simulink model "task1"  (R2024a)
settings: Solver=VariableStepAuto  StartTime=0.0  StopTime=10.0  MaxStep=0.01  RelTol=1e-3
undefined symbols (not defined in the file): A, B, Bf, CZ, G, K1, K2, wf0, x0
settings Model: Creator=sizgr  LastModifiedBy=sizgr

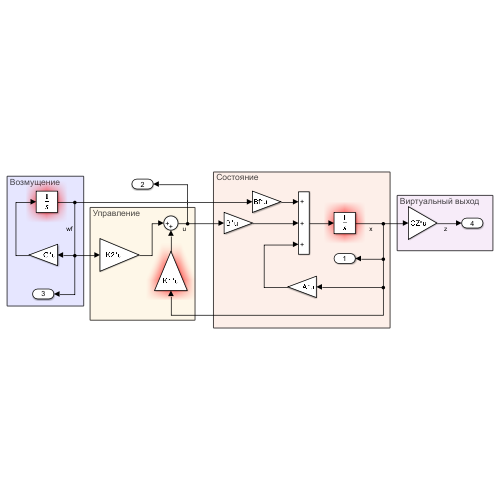
[thumbnail: Simulink's stored preview of the top-level diagram]
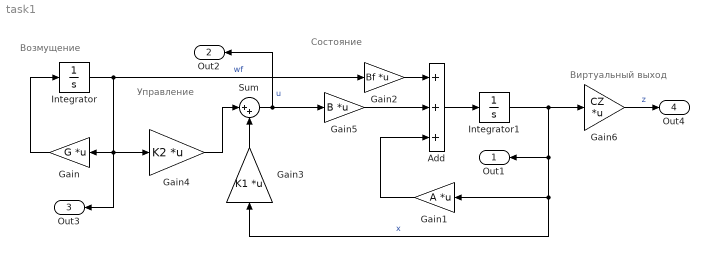
== system task1 ==
  note: Состояние
  note: Виртуальный выход
  note: Управление
  note: Возмущение
  Add : Sum  Inputs=+++
  Gain : Gain  Gain=G  Multiplication=Matrix(K*u)
  Gain1 : Gain  Gain=A  Multiplication=Matrix(K*u)
  Gain2 : Gain  Gain=Bf  Multiplication=Matrix(K*u)
  Gain3 : Gain  Gain=K1  Multiplication=Matrix(K*u)
  Gain4 : Gain  Gain=K2  Multiplication=Matrix(K*u)
  Gain5 : Gain  Gain=B  Multiplication=Matrix(K*u)
  Gain6 : Gain  Gain=CZ  Multiplication=Matrix(K*u)
  Integrator : Integrator  InitialCondition=wf0
  Integrator1 : Integrator  InitialCondition=x0
  Sum : Sum  Inputs=|++
  Out1 : Outport
  Out2 : Outport  Port=2
  Out3 : Outport  Port=3
  Out4 : Outport  Port=4
  wires:
  Integrator/1 -> Out3/1, Gain/1, Gain4/1, Gain2/1  "wf"
  Gain/1 -> Integrator/1
  Integrator1/1 -> Out1/1, Gain1/1, Gain3/1, Gain6/1  "x"
  Gain1/1 -> Add/3
  Add/1 -> Integrator1/1
  Gain2/1 -> Add/1
  Gain4/1 -> Sum/1
  Gain3/1 -> Sum/2
  Sum/1 -> Out2/1, Gain5/1  "u"
  Gain5/1 -> Add/2
  Gain6/1 -> Out4/1  "z"
